simulink model "dystonia_emg"  (Simulink 7.8)
settings: Solver=ode2  StartTime=0.0  StopTime=10  FixedStep=T  RelTol=1e-3
InitFcn:
  | [A tau T] = emg_filter();
  | 
  | 
  | %data = load('C:\Users\PXI_BBDL\Desktop\SfN2012\reflex_normal_0000.txt');
  | %data = data(2162:end , :);
  | %data = load('C:\Users\PXI_BBDL\Desktop\SfN2012\reflex_dystonia_2264_2648.txt');
  | %data = data( : , :);
  | %data = load('C:\Users\PXI_BBDL\Desktop\SfN2012\sine_nodystonia.txt');
  | %data = data(4200:end , :);
  | data = load('C:\Users\PXI_BBDL\Desktop\SfN2012\sine_yesdystonia.txt');
  | data = data(3600:end , :);
  | time = data(:, 1) - data(1,1);
  | MN_spkcnt_bic = [time data(:, 5)];
  | MN_spkcnt_tri = [time data(:, 5+4)];
  | 
  | lce_bic = [time data(:, 2)];
  | lce_tri = [time data(:, 2+4)];
  | 
  | force_bic = [time data(:, 4)];
  | force_tri = [time data(:, 4+4)];
StopFcn:
  | %recruitment_pattern_plotter(spikes_g1, spikes_g2, total_force, 0.02)
  | incrementVars('dystonia_emg')
values from neighbouring files (symbols this model uses):
  A = exp(-T/tau)    [emg_filter.m]    (also in twitch_filter.m = [1 -2*A_twitch A_twitch^2] * P * e * A_twitch / tau_twitch)
  T = 1/1024    (= 0.0009765625)    [emg_filter.m]    (also in get_active_function_coeff.m = 0.001; set_mu.m = 0.001; set_mu_spasticity.m = 0.001; set_trfcn.m = 0.001)
  tau = 0.008    [emg_filter.m]
undefined symbols (not defined in the file or in its folder): dfilt, fdesignblkfcn, gcbh
libraries: dsparch4 x7, cstblocks x1
settings Model: Creator=minos_niu  LastModifiedBy=PXI_BBDL

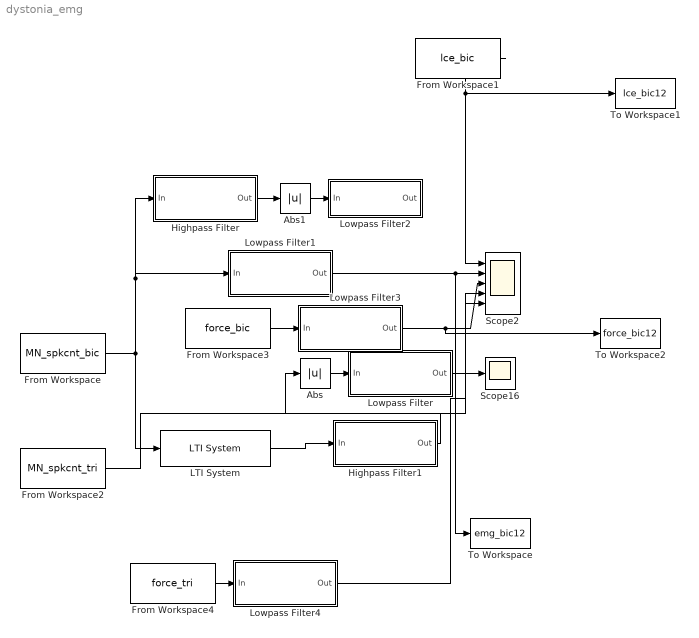
== system dystonia_emg ==
  Abs : Abs
  Abs1 : Abs
  From Workspace : FromWorkspace  VariableName=MN_spkcnt_bic  SampleTime=T
  From Workspace1 : FromWorkspace  VariableName=lce_bic  SampleTime=T
  From Workspace2 : FromWorkspace  VariableName=MN_spkcnt_tri  SampleTime=T
  From Workspace3 : FromWorkspace  VariableName=force_bic  SampleTime=T
  From Workspace4 : FromWorkspace  VariableName=force_tri  SampleTime=T
  Highpass Filter : Subsystem  DialogController=fdesignblkfcn  DialogControllerArgs=DataTag1  InitFcn=fdesignblkfcn(gcbh, {'InitFcn'});
      settings: CopyFcn=fdesignblkfcn(gcbh, {'CopyFcn'});
      mask Type: Highpass Filter
      mask Description: Design a highpass filter
      mask Help: helpview(mapfilelocation('dsp'), 'dsphighpassfilter');
      mask Display: disp('Highpass')
  Highpass Filter1 : Subsystem  DialogController=fdesignblkfcn  DialogControllerArgs=DataTag4  InitFcn=fdesignblkfcn(gcbh, {'InitFcn'});
      settings: CopyFcn=fdesignblkfcn(gcbh, {'CopyFcn'});
      mask Type: Highpass Filter
      mask Description: Design a highpass filter
      mask Help: helpview(mapfilelocation('dsp'), 'dsphighpassfilter');
      mask Display: disp('Highpass')
  LTI System : cstblocks/LTI System  sys=zpk([0], [A A], 2*T*A, T) - zpk([0 -A], [A A A], T^2*A/tau, T)  IC=[]
  Lowpass Filter : Subsystem  DialogController=fdesignblkfcn  DialogControllerArgs=DataTag7  InitFcn=fdesignblkfcn(gcbh, {'InitFcn'});
      settings: CopyFcn=fdesignblkfcn(gcbh, {'CopyFcn'});
      mask Type: Lowpass Filter
      mask Description: Design a lowpass filter
      mask Help: helpview(mapfilelocation('dsp'), 'dsplowpassfilter');
      mask Display: disp('Lowpass')
  Lowpass Filter1 : Subsystem  DialogController=fdesignblkfcn  DialogControllerArgs=DataTag10  InitFcn=fdesignblkfcn(gcbh, {'InitFcn'});
      settings: CopyFcn=fdesignblkfcn(gcbh, {'CopyFcn'});
      mask Type: Lowpass Filter
      mask Description: Design a lowpass filter
      mask Help: helpview(mapfilelocation('dsp'), 'dsplowpassfilter');
      mask Display: disp('Lowpass')
  Lowpass Filter2 : Subsystem  DialogController=fdesignblkfcn  DialogControllerArgs=DataTag13  InitFcn=fdesignblkfcn(gcbh, {'InitFcn'});
      settings: CopyFcn=fdesignblkfcn(gcbh, {'CopyFcn'});
      mask Type: Lowpass Filter
      mask Description: Design a lowpass filter
      mask Help: helpview(mapfilelocation('dsp'), 'dsplowpassfilter');
      mask Display: disp('Lowpass')
  Lowpass Filter3 : Subsystem  DialogController=fdesignblkfcn  DialogControllerArgs=DataTag16  InitFcn=fdesignblkfcn(gcbh, {'InitFcn'});
      settings: CopyFcn=fdesignblkfcn(gcbh, {'CopyFcn'});
      mask Type: Lowpass Filter
      mask Description: Design a lowpass filter
      mask Help: helpview(mapfilelocation('dsp'), 'dsplowpassfilter');
      mask Display: disp('Lowpass')
  Lowpass Filter4 : Subsystem  DialogController=fdesignblkfcn  DialogControllerArgs=DataTag19  InitFcn=fdesignblkfcn(gcbh, {'InitFcn'});
      settings: CopyFcn=fdesignblkfcn(gcbh, {'CopyFcn'});
      mask Type: Lowpass Filter
      mask Description: Design a lowpass filter
      mask Help: helpview(mapfilelocation('dsp'), 'dsplowpassfilter');
      mask Display: disp('Lowpass')
  Scope16 : Scope
      settings: TimeRange=10  YMin=0  YMax=350000  SaveName=total_force  DataFormat=Structure
  Scope2 : Scope  NumInputPorts=5
      settings: TimeRange=3  YMin=0.9~-0.5~-5~-5~-5  YMax=1.4~1~5~5~5  SaveName=total_force1  DataFormat=Structure
  To Workspace : ToWorkspace  VariableName=emg_bic12  SampleTime=-1  SaveFormat=Structure With Time
  To Workspace1 : ToWorkspace  VariableName=lce_bic12  SampleTime=-1  SaveFormat=Structure With Time
  To Workspace2 : ToWorkspace  VariableName=force_bic12  SampleTime=-1  SaveFormat=Structure With Time
  wires:
  Lowpass Filter/1(Out) -> Scope16/1
  LTI System/1 -> Highpass Filter1/1(In)
  From Workspace/1 -> LTI System/1, Highpass Filter/1(In), Lowpass Filter1/1(In)
  Abs/1 -> Lowpass Filter/1(In)
  From Workspace1/1 -> Scope2/1, To Workspace1/1
  Highpass Filter/1(Out) -> Abs1/1
  Abs1/1 -> Lowpass Filter2/1(In)
  Highpass Filter1/1(Out) -> Abs/1
  From Workspace3/1 -> Lowpass Filter3/1(In)
  Lowpass Filter3/1(Out) -> Scope2/3, To Workspace2/1
  From Workspace4/1 -> Lowpass Filter4/1(In)
  Lowpass Filter4/1(Out) -> Scope2/5
  From Workspace2/1 -> Scope2/4
  Lowpass Filter1/1(Out) -> Scope2/2, To Workspace/1

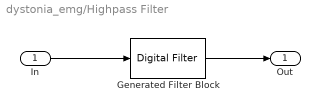
== system dystonia_emg/Highpass Filter ==
  In : Inport
  Generated Filter Block : dsparch4/Digital Filter  Tag=BlockMethodSubSystem  TypePopup=FIR (all zeros)  IIRFiltStruct=Direct form II transposed  AllPoleFiltStruct=Direct form  FIRFiltStruct=Direct form  CoeffSource=Specify via dialog  NumCoeffs=[-0.00171368266511031 0.00831437844808058 -0.0127173552334869 0.00556095179025038 0.00733971024255362 -0.00653104905017926 -0.0076900499697795 0.00902698316809851 0.00883886189950909 -0.0129607413537662 -0.0100749586672528 0.0185201740100089 0.0112333546135889 -0.0263752483836136 -0.0122707821857659 0.0381809766923897 0.0131304259182936 -0.0582933593251923 -0.0137682959486481 0.102813257992074 0.0141678767738541 -0.317202552416035 0.485698046170518 -0.317202552416035 0.0141678767738541 0.102813257992074 -0.0137682959486481 -0.0582933593251923 0.0131304259182936 0.0381809766923897 -0.0122707821857659 -0.0263752483836136 0.0112333546135889 0.0185201740100089 -0.0100749586672528 -0.0129607413537662 0.00883886189950909 0.00902698316809851 -0.0076900499697795 -0.00653104905017926 0.00733971024255362 0.00556095179025038 -0.0127173552334869 0.00831437844808058 -0.00171368266511031]  DenCoeffs=[1 0.1]  BiQuadCoeffs=[1 0.3 0.4 1 0.1 0.2]  LatticeCoeffs=[0.2 0.4]  denIgnore=on  FiltPerSampPopup=One filter per frame  IC=0  ICnum=0  ICden=0  roundingMode=Floor  overflowMode=off  ScaleValues=1  scaleValueFracLength=14  stageInFracLength=15  stageOutFracLength=15  FilterSource=Specify via dialog  dfiltObjectName=dfilt.dffir([1 2 1])  InputProcessing=Columns as channels (frame based)
  Out : Outport
  wires:
  Generated Filter Block/1 -> Out/1
  In/1 -> Generated Filter Block/1

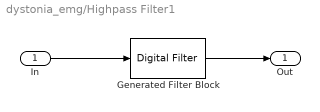
== system dystonia_emg/Highpass Filter1 ==
  In : Inport
  Generated Filter Block : dsparch4/Digital Filter  Tag=BlockMethodSubSystem  TypePopup=FIR (all zeros)  IIRFiltStruct=Direct form II transposed  AllPoleFiltStruct=Direct form  FIRFiltStruct=Direct form  CoeffSource=Specify via dialog  NumCoeffs=[-0.00171368266511031 0.00831437844808058 -0.0127173552334869 0.00556095179025038 0.00733971024255362 -0.00653104905017926 -0.0076900499697795 0.00902698316809851 0.00883886189950909 -0.0129607413537662 -0.0100749586672528 0.0185201740100089 0.0112333546135889 -0.0263752483836136 -0.0122707821857659 0.0381809766923897 0.0131304259182936 -0.0582933593251923 -0.0137682959486481 0.102813257992074 0.0141678767738541 -0.317202552416035 0.485698046170518 -0.317202552416035 0.0141678767738541 0.102813257992074 -0.0137682959486481 -0.0582933593251923 0.0131304259182936 0.0381809766923897 -0.0122707821857659 -0.0263752483836136 0.0112333546135889 0.0185201740100089 -0.0100749586672528 -0.0129607413537662 0.00883886189950909 0.00902698316809851 -0.0076900499697795 -0.00653104905017926 0.00733971024255362 0.00556095179025038 -0.0127173552334869 0.00831437844808058 -0.00171368266511031]  DenCoeffs=[1 0.1]  BiQuadCoeffs=[1 0.3 0.4 1 0.1 0.2]  LatticeCoeffs=[0.2 0.4]  denIgnore=on  FiltPerSampPopup=One filter per frame  IC=0  ICnum=0  ICden=0  roundingMode=Floor  overflowMode=off  ScaleValues=1  scaleValueFracLength=14  stageInFracLength=15  stageOutFracLength=15  FilterSource=Specify via dialog  dfiltObjectName=dfilt.dffir([1 2 1])  InputProcessing=Columns as channels (frame based)
  Out : Outport
  wires:
  In/1 -> Generated Filter Block/1
  Generated Filter Block/1 -> Out/1

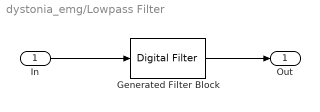
== system dystonia_emg/Lowpass Filter ==
  In : Inport
  Generated Filter Block : dsparch4/Digital Filter  Tag=BlockMethodSubSystem  TypePopup=FIR (all zeros)  IIRFiltStruct=Direct form II transposed  AllPoleFiltStruct=Direct form  FIRFiltStruct=Direct form  CoeffSource=Specify via dialog  NumCoeffs=[0.000789718777857514 0.000744577185831723 0.00107823000044434 0.00149476404221054 0.00200269045724713 0.00261008369831054 0.0033235203243232 0.00414853075427835 0.00508827739764678 0.00614377649471276 0.00731330348155772 0.00859334926052174 0.00997698249763242 0.0114554208341836 0.0130152727646894 0.0146425260653287 0.0163190525907415 0.0180261734331552 0.0197413015259351 0.0214414865019549 0.0231028765340779 0.0247019481907321 0.0262120529346396 0.0276110315008728 0.0288758696321162 0.0299846212957695 0.0309198615981866 0.0316640697639878 0.0322055579489813 0.0325340736126983 0.0326444214533691 0.0325340736126983 0.0322055579489813 0.0316640697639878 0.0309198615981866 0.0299846212957695 0.0288758696321162 0.0276110315008728 0.0262120529346396 0.0247019481907321 0.0231028765340779 0.0214414865019549 0.0197413015259351 0.0180261734331552 0.0163190525907415 0.0146425260653287 0.0130152727646894 0.0114554208341836 0.00997698249763242 0.00859334926052174 0.00731330348155772 0.00614377649471276 0.00508827739764678 0.00414853075427835 0.0033235203243232 0.00261008369831054 0.00200269045724713 0.00149476404221054 0.00107823000044434 0.000744577185831723 0.000789718777857514]  DenCoeffs=[1 0.1]  BiQuadCoeffs=[1 0.3 0.4 1 0.1 0.2]  LatticeCoeffs=[0.2 0.4]  denIgnore=on  FiltPerSampPopup=One filter per frame  IC=0  ICnum=0  ICden=0  roundingMode=Floor  overflowMode=off  ScaleValues=1  scaleValueFracLength=14  stageInFracLength=15  stageOutFracLength=15  FilterSource=Specify via dialog  dfiltObjectName=dfilt.dffir([1 2 1])  InputProcessing=Columns as channels (frame based)
  Out : Outport
  wires:
  Generated Filter Block/1 -> Out/1
  In/1 -> Generated Filter Block/1

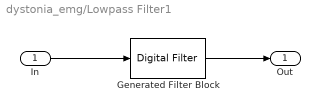
== system dystonia_emg/Lowpass Filter1 ==
  In : Inport
  Generated Filter Block : dsparch4/Digital Filter  Tag=BlockMethodSubSystem  TypePopup=FIR (all zeros)  IIRFiltStruct=Direct form II transposed  AllPoleFiltStruct=Direct form  FIRFiltStruct=Direct form  CoeffSource=Specify via dialog  NumCoeffs=[0.00239420808341765 0.00790188746065433 0.0184933235577627 0.0348472274262868 0.0561245897493372 0.0796407261947382 0.101287735410592 0.116603816509964 0.122140868395091 0.116603816509964 0.101287735410592 0.0796407261947382 0.0561245897493372 0.0348472274262868 0.0184933235577627 0.00790188746065433 0.00239420808341765]  DenCoeffs=[1 0.1]  BiQuadCoeffs=[1 0.3 0.4 1 0.1 0.2]  LatticeCoeffs=[0.2 0.4]  denIgnore=on  FiltPerSampPopup=One filter per frame  IC=0  ICnum=0  ICden=0  roundingMode=Floor  overflowMode=off  ScaleValues=1  scaleValueFracLength=14  stageInFracLength=15  stageOutFracLength=15  FilterSource=Specify via dialog  dfiltObjectName=dfilt.dffir([1 2 1])  InputProcessing=Columns as channels (frame based)
  Out : Outport
  wires:
  Generated Filter Block/1 -> Out/1
  In/1 -> Generated Filter Block/1

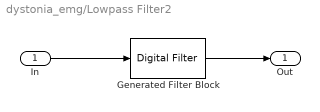
== system dystonia_emg/Lowpass Filter2 ==
  In : Inport
  Generated Filter Block : dsparch4/Digital Filter  Tag=BlockMethodSubSystem  TypePopup=FIR (all zeros)  IIRFiltStruct=Direct form II transposed  AllPoleFiltStruct=Direct form  FIRFiltStruct=Direct form  CoeffSource=Specify via dialog  NumCoeffs=[0.000979821768041705 0.00137738938209103 0.0022721888505315 0.00347582631381654 0.0050261219451391 0.00695078539042112 0.00926295711622131 0.0119590396023665 0.0150149295577601 0.0183861354850592 0.0220068142303519 0.0257929847976959 0.0296427358301452 0.0334414793011898 0.0370673735172187 0.0403980382619209 0.0433134164957781 0.0457057282231088 0.0474846740757913 0.0485805615376401 0.0489507228120537 0.0485805615376401 0.0474846740757913 0.0457057282231088 0.0433134164957781 0.0403980382619209 0.0370673735172187 0.0334414793011898 0.0296427358301452 0.0257929847976959 0.0220068142303519 0.0183861354850592 0.0150149295577601 0.0119590396023665 0.00926295711622131 0.00695078539042112 0.0050261219451391 0.00347582631381654 0.0022721888505315 0.00137738938209103 0.000979821768041705]  DenCoeffs=[1 0.1]  BiQuadCoeffs=[1 0.3 0.4 1 0.1 0.2]  LatticeCoeffs=[0.2 0.4]  denIgnore=on  FiltPerSampPopup=One filter per frame  IC=0  ICnum=0  ICden=0  roundingMode=Floor  overflowMode=off  ScaleValues=1  scaleValueFracLength=14  stageInFracLength=15  stageOutFracLength=15  FilterSource=Specify via dialog  dfiltObjectName=dfilt.dffir([1 2 1])  InputProcessing=Columns as channels (frame based)
  Out : Outport
  wires:
  In/1 -> Generated Filter Block/1
  Generated Filter Block/1 -> Out/1

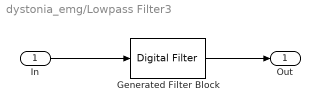
== system dystonia_emg/Lowpass Filter3 ==
  In : Inport
  Generated Filter Block : dsparch4/Digital Filter  Tag=BlockMethodSubSystem  TypePopup=FIR (all zeros)  IIRFiltStruct=Direct form II transposed  AllPoleFiltStruct=Direct form  FIRFiltStruct=Direct form  CoeffSource=Specify via dialog  NumCoeffs=[0.000979821768041705 0.00137738938209103 0.0022721888505315 0.00347582631381654 0.0050261219451391 0.00695078539042112 0.00926295711622131 0.0119590396023665 0.0150149295577601 0.0183861354850592 0.0220068142303519 0.0257929847976959 0.0296427358301452 0.0334414793011898 0.0370673735172187 0.0403980382619209 0.0433134164957781 0.0457057282231088 0.0474846740757913 0.0485805615376401 0.0489507228120537 0.0485805615376401 0.0474846740757913 0.0457057282231088 0.0433134164957781 0.0403980382619209 0.0370673735172187 0.0334414793011898 0.0296427358301452 0.0257929847976959 0.0220068142303519 0.0183861354850592 0.0150149295577601 0.0119590396023665 0.00926295711622131 0.00695078539042112 0.0050261219451391 0.00347582631381654 0.0022721888505315 0.00137738938209103 0.000979821768041705]  DenCoeffs=[1 0.1]  BiQuadCoeffs=[1 0.3 0.4 1 0.1 0.2]  LatticeCoeffs=[0.2 0.4]  denIgnore=on  FiltPerSampPopup=One filter per frame  IC=0  ICnum=0  ICden=0  roundingMode=Floor  overflowMode=off  ScaleValues=1  scaleValueFracLength=14  stageInFracLength=15  stageOutFracLength=15  FilterSource=Specify via dialog  dfiltObjectName=dfilt.dffir([1 2 1])  InputProcessing=Columns as channels (frame based)
  Out : Outport
  wires:
  Generated Filter Block/1 -> Out/1
  In/1 -> Generated Filter Block/1

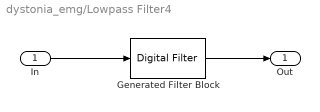
== system dystonia_emg/Lowpass Filter4 ==
  In : Inport
  Generated Filter Block : dsparch4/Digital Filter  Tag=BlockMethodSubSystem  TypePopup=FIR (all zeros)  IIRFiltStruct=Direct form II transposed  AllPoleFiltStruct=Direct form  FIRFiltStruct=Direct form  CoeffSource=Specify via dialog  NumCoeffs=[0.000979821768041705 0.00137738938209103 0.0022721888505315 0.00347582631381654 0.0050261219451391 0.00695078539042112 0.00926295711622131 0.0119590396023665 0.0150149295577601 0.0183861354850592 0.0220068142303519 0.0257929847976959 0.0296427358301452 0.0334414793011898 0.0370673735172187 0.0403980382619209 0.0433134164957781 0.0457057282231088 0.0474846740757913 0.0485805615376401 0.0489507228120537 0.0485805615376401 0.0474846740757913 0.0457057282231088 0.0433134164957781 0.0403980382619209 0.0370673735172187 0.0334414793011898 0.0296427358301452 0.0257929847976959 0.0220068142303519 0.0183861354850592 0.0150149295577601 0.0119590396023665 0.00926295711622131 0.00695078539042112 0.0050261219451391 0.00347582631381654 0.0022721888505315 0.00137738938209103 0.000979821768041705]  DenCoeffs=[1 0.1]  BiQuadCoeffs=[1 0.3 0.4 1 0.1 0.2]  LatticeCoeffs=[0.2 0.4]  denIgnore=on  FiltPerSampPopup=One filter per frame  IC=0  ICnum=0  ICden=0  roundingMode=Floor  overflowMode=off  ScaleValues=1  scaleValueFracLength=14  stageInFracLength=15  stageOutFracLength=15  FilterSource=Specify via dialog  dfiltObjectName=dfilt.dffir([1 2 1])  InputProcessing=Columns as channels (frame based)
  Out : Outport
  wires:
  In/1 -> Generated Filter Block/1
  Generated Filter Block/1 -> Out/1
